simulink model "Pulse_Control_Signal"  (R2022b)
settings: Solver=VariableStepAuto  StartTime=0.0  StopTime=0.9  RelTol=1e-3
settings Model: Creator=Rio  LastModifiedBy=Rio

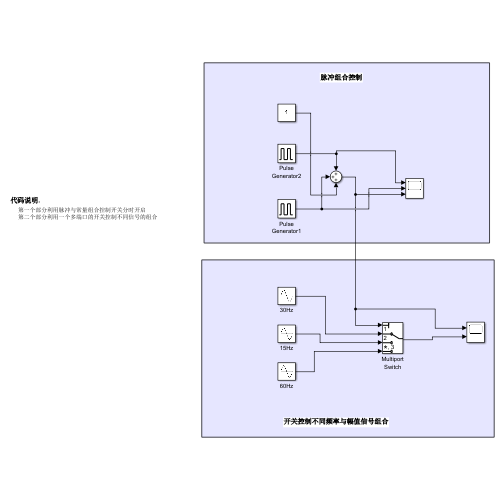
[thumbnail: Simulink's stored preview of the top-level diagram]
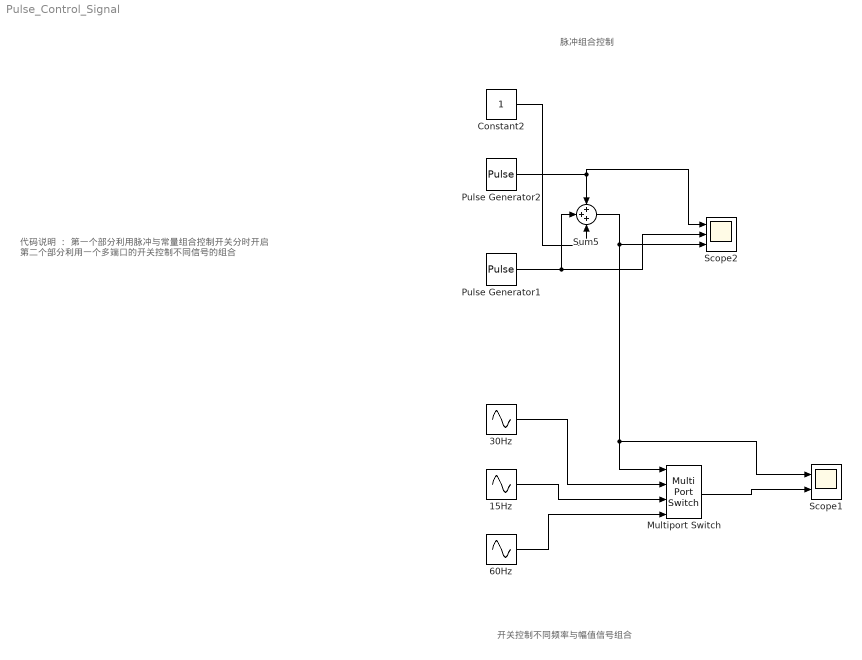
== system Pulse_Control_Signal ==
  note: 脉冲组合控制
  note: 代码说明 ：
      | 第一个部分利用脉冲与常量组合控制开关分时开启
      | 第二个部分利用一个多端口的开关控制不同信号的组合
  note: 开关控制不同频率与幅值信号组合
  15Hz : Sin  Amplitude=1.5*1  Frequency=2*pi*15  SampleTime=0
  30Hz : Sin  Frequency=2*pi*30  SampleTime=0
  60Hz : Sin  Amplitude=0.6*1  Frequency=2*pi*60  SampleTime=0
  Constant2 : Constant
  Multiport Switch : MultiPortSwitch  SaturateOnIntegerOverflow=off  InputSameDT=off
  Pulse Generator1 : DiscretePulseGenerator  PulseType=Time based  Amplitude=2  Period=0.9  PulseWidth=100/3
  Pulse Generator2 : DiscretePulseGenerator  PulseType=Time based  Period=0.9  PulseWidth=100/3  PhaseDelay=0.3
  Scope1 : Scope  NumInputPorts=2
  Scope2 : Scope  NumInputPorts=3
  Sum5 : Sum  Inputs=+++
  wires:
  Constant2/1 -> Sum5/3
  Pulse Generator2/1 -> Scope2/1, Sum5/1
  Pulse Generator1/1 -> Sum5/2, Scope2/2
  30Hz/1 -> Multiport Switch/2
  60Hz/1 -> Multiport Switch/4
  15Hz/1 -> Multiport Switch/3
  Sum5/1 -> Multiport Switch/1, Scope1/1, Scope2/3
  Multiport Switch/1 -> Scope1/2
